simulink model "fsm_12B_with_contracts_SLDV"  (R2019b)
settings: Solver=FixedStepDiscrete  StartTime=0.0  StopTime=10  RelTol=1e-3  EnableMultiTasking=on
model workspace (MAT data in the model file):
  ContractValidatorBlocksMap : containers.Map (value not decoded)
libraries: sldvlib x20, cocosimLibs x20
(part 1 of 2)
settings Model: Creator=elliocm  LastModifiedBy=hbourbou
settings DataIOCC: LimitDataPoints=on  SaveFormat=Array  ReturnWorkspaceOutputs=off
settings OptimizationCC: ExpressionDepthLimit=2147483647  LifeSpan=inf
settings DebuggingCC: UnderspecifiedInitializationDetection=Classic  MergeDetectMultiDrivingBlocksExec=none  SolverPrmCheckMsg=warning  StateNameClashWarn=warning  SFUnexpectedBacktrackingDiag=warning  SFNoUnconditionalDefaultTransitionDiag=warning  SFExecutionAtInitializationDiag=none  ArithmeticOperatorsInVariantConditions=warning
settings HardwareCC: ProdBitPerPointer=32  ProdBitPerSizeT=32  ProdBitPerPtrDiffT=32  ProdLargestAtomicFloat=None  ProdIntDivRoundTo=Undefined  ProdEndianess=Unspecified  ProdWordSize=32  ProdHWDeviceType=32-bit Generic
settings ModelReferenceCC: PropagateSignalLabelsOutOfModel=off
settings SFSimCC: SimUseLocalCustomCode=off  CustomCodeUndefinedFunction=UseInterfaceOnly
settings RTWCC: RTWUseLocalCustomCode=off
settings CodeAppCC: StateflowObjectComments=on
settings GRTTargetCC: TargetLangStandard=C89/C90 (ANSI)  GeneratePreprocessorConditionals=Disable all
settings ConfigComp: CovMetricSettings=dw  CovHtmlReporting=on  CovSaveCumulativeToWorkspaceVar=on  CovSaveSingleToWorkspaceVar=on  CovExternalEMLEnable=off  DVMode=PropertyProving  DVTestSuiteOptimization=Auto  DVDetectOutOfBounds=on

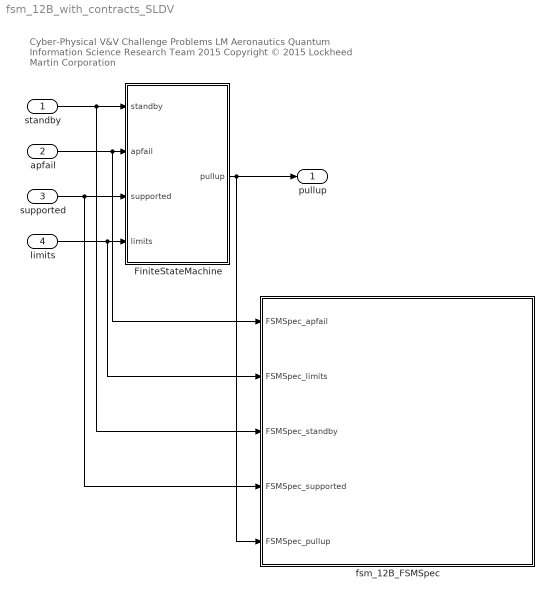
== system fsm_12B_with_contracts_SLDV ==
  note: Cyber-Physical V&V Challenge Problems
      | LM Aeronautics Quantum Information Science Research Team 2015
      | Copyright © 2015 Lockheed Martin Corporation
  standby : Inport  OutDataTypeStr=boolean
  apfail : Inport  Port=2  OutDataTypeStr=boolean
  supported : Inport  Port=3  OutDataTypeStr=boolean
  limits : Inport  Port=4  OutDataTypeStr=boolean
  FiniteStateMachine : Subsystem
  fsm_12B_FSMSpec : Subsystem  TreatAsAtomicUnit=on  SimViewingDevice=on  mask(VerificationSubsystem){}
      mask Display: image(imread('sldvicon_versubsys.png','BackGroundColor',[1 1 1]),'center');
  pullup : Outport  VectorParamsAs1DForOutWhenUnconnected=off
  wires:
  standby/1 -> FiniteStateMachine/1(standby), fsm_12B_FSMSpec/3(FSMSpec_standby)
  apfail/1 -> FiniteStateMachine/2(apfail), fsm_12B_FSMSpec/1(FSMSpec_apfail)
  supported/1 -> FiniteStateMachine/3(supported), fsm_12B_FSMSpec/4(FSMSpec_supported)
  limits/1 -> FiniteStateMachine/4(limits), fsm_12B_FSMSpec/2(FSMSpec_limits)
  FiniteStateMachine/1(pullup) -> pullup/1, fsm_12B_FSMSpec/5(FSMSpec_pullup)

== system fsm_12B_with_contracts_SLDV/FiniteStateMachine ==
  note: 51
  standby : Inport
  apfail : Inport  Port=2
  supported : Inport  Port=3
  limits : Inport  Port=4
  FiniteStateMachine_FSM_AutopilotSpec1 : Subsystem  TreatAsAtomicUnit=on  SimViewingDevice=on  mask(VerificationSubsystem){}
      mask Display: image(imread('sldvicon_versubsys.png','BackGroundColor',[1 1 1]),'center');
  FiniteStateMachine_FSM_SensorSpec : Subsystem  TreatAsAtomicUnit=on  SimViewingDevice=on  mask(VerificationSubsystem){}
      mask Display: image(imread('sldvicon_versubsys.png','BackGroundColor',[1 1 1]),'center');
  Manager : Subsystem
  Sen : Subsystem
  Unit Delay : UnitDelay  SampleTime=-1  HasFrameUpgradeWarning=on
  Unit Delay1 : UnitDelay  SampleTime=-1  HasFrameUpgradeWarning=on
  Unit Delay2 : UnitDelay  InitialCondition=1  SampleTime=-1  HasFrameUpgradeWarning=on
  pullup : Outport  VectorParamsAs1DForOutWhenUnconnected=off
  wires:
  Manager/1(MODE) -> FiniteStateMachine_FSM_SensorSpec/1(FSM_SensorSpec_MODE), Sen/1(mode)
  Manager/4(STATE) -> FiniteStateMachine_FSM_AutopilotSpec1/6(FSM_AutopilotSpec_STATE), Unit Delay/1
  Unit Delay/1 -> FiniteStateMachine_FSM_AutopilotSpec1/4(FSM_AutopilotSpec_state), Manager/5(state)
  Manager/2(REQUEST) -> FiniteStateMachine_FSM_SensorSpec/3(FSM_SensorSpec_request), Sen/2(request)
  Unit Delay1/1 -> FiniteStateMachine_FSM_SensorSpec/4(FSM_SensorSpec_senstate), Sen/4(senstate)
  Unit Delay2/1 -> FiniteStateMachine_FSM_AutopilotSpec1/2(FSM_AutopilotSpec_good), Manager/4(good)
  Sen/2(SENSTATE) -> FiniteStateMachine_FSM_SensorSpec/5(FSM_SensorSpec_SENSTATE), Unit Delay1/1
  Sen/1(good) -> Unit Delay2/1
  Manager/3(PULL) -> pullup/1
  standby/1 -> FiniteStateMachine_FSM_AutopilotSpec1/3(FSM_AutopilotSpec_standby), Manager/1(standby)
  apfail/1 -> FiniteStateMachine_FSM_AutopilotSpec1/1(FSM_AutopilotSpec_apfail), Manager/2(apfail)
  supported/1 -> FiniteStateMachine_FSM_AutopilotSpec1/5(FSM_AutopilotSpec_supported), Manager/3(supported)
  limits/1 -> Sen/3(limits), FiniteStateMachine_FSM_SensorSpec/2(FSM_SensorSpec_limits)

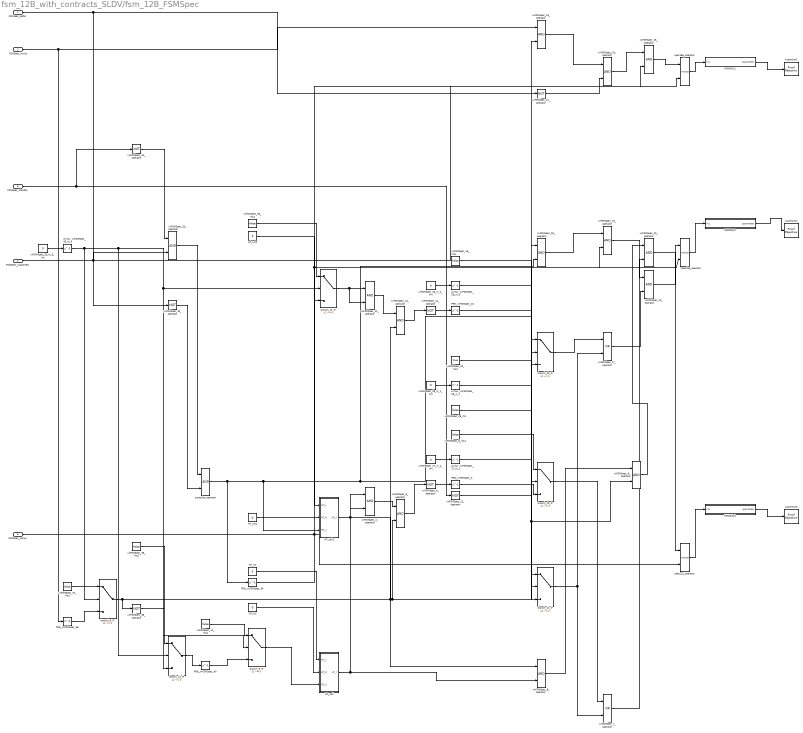
== system fsm_12B_with_contracts_SLDV/fsm_12B_FSMSpec ==
  FSMSpec_apfail : Inport  OutDataTypeStr=boolean
  FSMSpec_limits : Inport  Port=2  OutDataTypeStr=boolean
  FSMSpec_standby : Inport  Port=3  OutDataTypeStr=boolean
  FSMSpec_supported : Inport  Port=4  OutDataTypeStr=boolean
  FSMSpec_pullup : Inport  Port=5  OutDataTypeStr=boolean
  Arrow_xxFSMSpec_26_ni_0 : Delay  DelayLength=1  InitialCondition=1
  Arrow_xxFSMSpec_27_ni_2 : Delay  DelayLength=1  InitialCondition=1
  Arrow_xxFSMSpec_28_ni_1 : Delay  DelayLength=1  InitialCondition=1
  Arrow_xxFSMSpec_33_ni_5 : Delay  DelayLength=1  InitialCondition=1
  Assertion1 : sldvlib/Objectives and Constraints/Proof Objective  enabled=on  customAVTBlockType=Proof Objective  intervals=true  dispValues=on  outEnabled=off  enableStopSim=off
      settings: AttributesFormatString=%<intervals>  SourceProductName=Simulink  SourceProductBaseCode=SL
  Assertion2 : sldvlib/Objectives and Constraints/Proof Objective  enabled=on  customAVTBlockType=Proof Objective  intervals=true  dispValues=on  outEnabled=off  enableStopSim=off
      settings: AttributesFormatString=%<intervals>  SourceProductName=Simulink  SourceProductBaseCode=SL
  Assertion3 : sldvlib/Objectives and Constraints/Proof Objective  enabled=on  customAVTBlockType=Proof Objective  intervals=true  dispValues=on  outEnabled=off  enableStopSim=off
      settings: AttributesFormatString=%<intervals>  SourceProductName=Simulink  SourceProductBaseCode=SL
  FSM001v1 : Subsystem
  FSM001v2 : Subsystem
  FSM001v3 : Subsystem
  HT_In1 : Constant  Value=3  OutDataTypeStr=int32
  HT_In11 : Constant  Value=3  OutDataTypeStr=int32
  HT_In2 : Constant  Value=0  OutDataTypeStr=int32
  HT_In21 : Constant  Value=0  OutDataTypeStr=int32
  HT_call : Subsystem
  HT_call1 : Subsystem
  PRE_xxFSMSpec_{5,15,34,36,40} (5 alike) : Delay  DelayLength=1  InitialCondition=0
  autopilot_operator : Logic  AllPortsSameDT=off  OutDataTypeStr=boolean
  branch_10_IF : Switch  Criteria=u2 ~= 0
  branch_11_IF : Switch  Criteria=u2 ~= 0
  branch_12_IF : Switch  Criteria=u2 ~= 0
  branch_13_IF : Switch  Criteria=u2 ~= 0
  branch_14_IF : Switch  Criteria=u2 ~= 0
  branch_8_IF : Switch  Criteria=u2 ~= 0
  branch_9_IF : Switch  Criteria=u2 ~= 0
  spec166_operator : cocosimLibs/Implies  SystemSampleTime=-1  Latency=0  AutoFrameSizeCalculation=off
  spec194_operator : cocosimLibs/Implies  SystemSampleTime=-1  Latency=0  AutoFrameSizeCalculation=off
  spec222_operator : cocosimLibs/Implies  SystemSampleTime=-1  Latency=0  AutoFrameSizeCalculation=off
  xxFSMSpec_10_operator : Logic  AllPortsSameDT=off  OutDataTypeStr=boolean
  xxFSMSpec_12_operator : Logic  AllPortsSameDT=off  OutDataTypeStr=boolean
  xxFSMSpec_13_operator : Logic  AllPortsSameDT=off  OutDataTypeStr=boolean
  xxFSMSpec_14_operator : Logic  Operator=NOT  AllPortsSameDT=off  OutDataTypeStr=boolean
  xxFSMSpec_16_rhs1 : Constant  Value=false  OutDataTypeStr=boolean
  xxFSMSpec_17_operator : Logic  Operator=OR  AllPortsSameDT=off  OutDataTypeStr=boolean
  xxFSMSpec_18_operator : Logic  AllPortsSameDT=off  OutDataTypeStr=boolean
  xxFSMSpec_19_operator : Logic  AllPortsSameDT=off  OutDataTypeStr=boolean
  xxFSMSpec_20_operator : Logic  AllPortsSameDT=off  OutDataTypeStr=boolean
  xxFSMSpec_21_operator : Logic  Operator=NOT  AllPortsSameDT=off  OutDataTypeStr=boolean
  xxFSMSpec_22_operator : Logic  Operator=NOT  AllPortsSameDT=off  OutDataTypeStr=boolean
  xxFSMSpec_23_operator : Logic  AllPortsSameDT=off  OutDataTypeStr=boolean
  xxFSMSpec_24_operator : Logic  AllPortsSameDT=off  OutDataTypeStr=boolean
  xxFSMSpec_25_operator : Logic  AllPortsSameDT=off  OutDataTypeStr=boolean
  xxFSMSpec_26_ni_0_init : Constant  Value=0  OutDataTypeStr=boolean
  xxFSMSpec_27_ni_2_init : Constant  Value=0  OutDataTypeStr=boolean
  xxFSMSpec_28_ni_1_init : Constant  Value=0  OutDataTypeStr=boolean
  xxFSMSpec_29_rhs : Constant  Value=false  OutDataTypeStr=boolean
  xxFSMSpec_29_rhs1 : Constant  Value=true  OutDataTypeStr=boolean
  xxFSMSpec_2_operator : Logic  AllPortsSameDT=off  OutDataTypeStr=boolean
  xxFSMSpec_30_operator : Logic  Operator=NOT  AllPortsSameDT=off  OutDataTypeStr=boolean
  xxFSMSpec_31_operator : Logic  Operator=NOT  AllPortsSameDT=off  OutDataTypeStr=boolean
  xxFSMSpec_32_operator : Logic  AllPortsSameDT=off  OutDataTypeStr=boolean
  xxFSMSpec_33_ni_5_init : Constant  Value=0  OutDataTypeStr=boolean
  xxFSMSpec_35_rhs1 : Constant  Value=false  OutDataTypeStr=boolean
  xxFSMSpec_37_rhs1 : Constant  Value=false  OutDataTypeStr=boolean
  xxFSMSpec_38_operator : Logic  Operator=NOT  AllPortsSameDT=off  OutDataTypeStr=boolean
  xxFSMSpec_39_rhs1 : Constant  Value=false  OutDataTypeStr=boolean
  xxFSMSpec_3_operator : Logic  AllPortsSameDT=off  OutDataTypeStr=boolean
  xxFSMSpec_41_rhs1 : Constant  Value=false  OutDataTypeStr=boolean
  xxFSMSpec_4_operator : Logic  Operator=NOT  AllPortsSameDT=off  OutDataTypeStr=boolean
  xxFSMSpec_6_rhs1 : Constant  Value=false  OutDataTypeStr=boolean
  xxFSMSpec_7_operator : Logic  Operator=OR  AllPortsSameDT=off  OutDataTypeStr=boolean
  xxFSMSpec_8_operator : Logic  AllPortsSameDT=off  OutDataTypeStr=boolean
  xxFSMSpec_9_operator : Logic  AllPortsSameDT=off  OutDataTypeStr=boolean
  wires:
  xxFSMSpec_8_operator/1 -> xxFSMSpec_9_operator/1
  branch_10_IF/1 -> xxFSMSpec_7_operator/1
  xxFSMSpec_3_operator/1 -> xxFSMSpec_4_operator/1
  xxFSMSpec_2_operator/1 -> xxFSMSpec_3_operator/1
  xxFSMSpec_31_operator/1 -> xxFSMSpec_32_operator/1
  xxFSMSpec_24_operator/1 -> xxFSMSpec_25_operator/1
  xxFSMSpec_21_operator/1 -> xxFSMSpec_24_operator/2
  xxFSMSpec_23_operator/1 -> xxFSMSpec_24_operator/1
  xxFSMSpec_22_operator/1 -> xxFSMSpec_23_operator/2
  xxFSMSpec_17_operator/1 -> xxFSMSpec_20_operator/2
  xxFSMSpec_19_operator/1 -> xxFSMSpec_20_operator/1
  xxFSMSpec_18_operator/1 -> xxFSMSpec_19_operator/1
  branch_13_IF/1 -> xxFSMSpec_17_operator/1
  xxFSMSpec_13_operator/1 -> xxFSMSpec_14_operator/1
  xxFSMSpec_12_operator/1 -> xxFSMSpec_13_operator/1
  xxFSMSpec_7_operator/1 -> xxFSMSpec_10_operator/2
  xxFSMSpec_9_operator/1 -> xxFSMSpec_10_operator/1
  xxFSMSpec_10_operator/1 -> spec222_operator/1
  xxFSMSpec_20_operator/1 -> spec194_operator/1
  xxFSMSpec_25_operator/1 -> spec166_operator/1
  spec222_operator/1 -> FSM001v3/1(In1)
  spec194_operator/1 -> FSM001v2/1(In1)
  spec166_operator/1 -> FSM001v1/1(In1)
  PRE_xxFSMSpec_40/1 -> branch_9_IF/3
  xxFSMSpec_41_rhs1/1 -> branch_9_IF/1
  PRE_xxFSMSpec_36/1 -> branch_8_IF/3
  xxFSMSpec_37_rhs1/1 -> branch_8_IF/1
  xxFSMSpec_38_operator/1 -> branch_14_IF/3
  xxFSMSpec_39_rhs1/1 -> branch_14_IF/1
  PRE_xxFSMSpec_15/1 -> branch_13_IF/3
  Arrow_xxFSMSpec_26_ni_0/1 -> branch_13_IF/2
  xxFSMSpec_16_rhs1/1 -> branch_13_IF/1
  PRE_xxFSMSpec_34/1 -> branch_12_IF/3
  xxFSMSpec_35_rhs1/1 -> branch_12_IF/1
  xxFSMSpec_29_rhs/1 -> branch_11_IF/3
  Arrow_xxFSMSpec_28_ni_1/1 -> branch_11_IF/2
  xxFSMSpec_29_rhs1/1 -> branch_11_IF/1
  PRE_xxFSMSpec_5/1 -> branch_10_IF/3
  Arrow_xxFSMSpec_27_ni_2/1 -> branch_10_IF/2
  xxFSMSpec_6_rhs1/1 -> branch_10_IF/1
  xxFSMSpec_30_operator/1 -> autopilot_operator/2
  xxFSMSpec_32_operator/1 -> autopilot_operator/1
  xxFSMSpec_4_operator/1 -> PRE_xxFSMSpec_5/1
  branch_14_IF/1 -> PRE_xxFSMSpec_40/1
  xxFSMSpec_14_operator/1 -> PRE_xxFSMSpec_15/1
  HT_In21/1 -> HT_call1/2(HT_R)
  HT_In11/1 -> HT_call1/1(HT_L)
  branch_9_IF/1 -> HT_call/3(HT_X)
  HT_In2/1 -> HT_call/2(HT_R)
  HT_In1/1 -> HT_call/1(HT_L)
  xxFSMSpec_33_ni_5_init/1 -> Arrow_xxFSMSpec_33_ni_5/1
  xxFSMSpec_28_ni_1_init/1 -> Arrow_xxFSMSpec_28_ni_1/1
  xxFSMSpec_27_ni_2_init/1 -> Arrow_xxFSMSpec_27_ni_2/1
  xxFSMSpec_26_ni_0_init/1 -> Arrow_xxFSMSpec_26_ni_0/1
  branch_8_IF/1 -> xxFSMSpec_9_operator/2, xxFSMSpec_19_operator/2, xxFSMSpec_3_operator/2, xxFSMSpec_13_operator/2, xxFSMSpec_38_operator/1
  branch_12_IF/1 -> xxFSMSpec_18_operator/2, xxFSMSpec_12_operator/2
  HT_call/1(HT_Y) -> xxFSMSpec_8_operator/2, xxFSMSpec_2_operator/2
  HT_call1/1(HT_Y) -> xxFSMSpec_8_operator/1, xxFSMSpec_2_operator/1
  FSMSpec_pullup/1 -> spec194_operator/2, spec166_operator/2, spec222_operator/2
  FSMSpec_supported/1 -> xxFSMSpec_32_operator/2, xxFSMSpec_25_operator/2
  FSMSpec_apfail/1 -> xxFSMSpec_30_operator/1, xxFSMSpec_21_operator/1
  FSMSpec_limits/1 -> xxFSMSpec_23_operator/1, PRE_xxFSMSpec_36/1
  FSMSpec_standby/1 -> xxFSMSpec_31_operator/1, xxFSMSpec_22_operator/1
  branch_11_IF/1 -> xxFSMSpec_7_operator/2, xxFSMSpec_17_operator/2
  Arrow_xxFSMSpec_33_ni_5/1 -> branch_9_IF/2, branch_12_IF/2, branch_14_IF/2, branch_8_IF/2
  autopilot_operator/1 -> xxFSMSpec_18_operator/1, xxFSMSpec_12_operator/1, HT_call1/3(HT_X), PRE_xxFSMSpec_34/1
  FSM001v1/1(guarantee) -> Assertion1/1
  FSM001v2/1(guarantee) -> Assertion2/1
  FSM001v3/1(guarantee) -> Assertion3/1

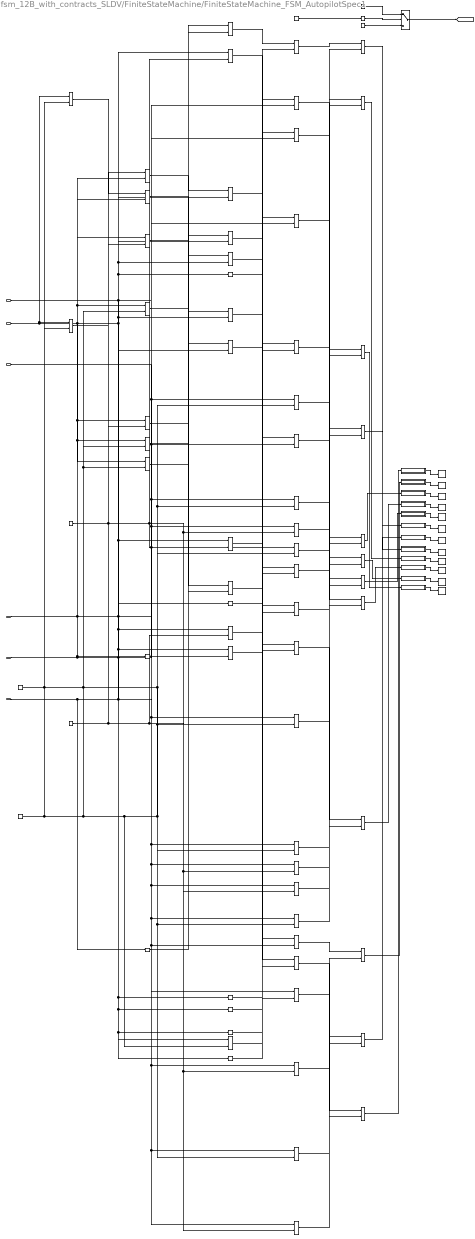
== system fsm_12B_with_contracts_SLDV/FiniteStateMachine/FiniteStateMachine_FSM_AutopilotSpec1 ==
  FSM_AutopilotSpec_apfail : Inport  OutDataTypeStr=boolean
  FSM_AutopilotSpec_good : Inport  Port=2  OutDataTypeStr=boolean
  FSM_AutopilotSpec_standby : Inport  Port=3  OutDataTypeStr=boolean
  FSM_AutopilotSpec_state : Inport  Port=4  OutDataTypeStr=double
  FSM_AutopilotSpec_supported : Inport  Port=5  OutDataTypeStr=boolean
  FSM_AutopilotSpec_STATE : Inport  Port=6  OutDataTypeStr=double
  Arrow_xxFSM_AutopilotSpec_54_ni_7 : Delay  DelayLength=1  InitialCondition=1
  Assertion{1..12} (12 alike) : sldvlib/Objectives and Constraints/Proof Objective  enabled=on  customAVTBlockType=Proof Objective  intervals=true  dispValues=on  outEnabled=off  enableStopSim=off
      settings: AttributesFormatString=%<intervals>  SourceProductName=Simulink  SourceProductBaseCode=SL
  FSM002 : Subsystem
  FSM003 : Subsystem
  FSM003v2 : Subsystem
  FSM004 : Subsystem
  FSM004v2 : Subsystem
  FSM005 : Subsystem
  FSM006 : Subsystem
  FSM007 : Subsystem
  FSM007v2 : Subsystem
  FSM008v1 : Subsystem
  FSM008v2 : Subsystem
  FSM009 : Subsystem
  branch_6_IF : Switch  Criteria=u2 ~= 0
  spec129_operator : cocosimLibs/Implies  SystemSampleTime=-1  Latency=0  AutoFrameSizeCalculation=off
  spec143_operator : cocosimLibs/Implies  SystemSampleTime=-1  Latency=0  AutoFrameSizeCalculation=off
  spec160_operator : cocosimLibs/Implies  SystemSampleTime=-1  Latency=0  AutoFrameSizeCalculation=off
  spec182_operator : cocosimLibs/Implies  SystemSampleTime=-1  Latency=0  AutoFrameSizeCalculation=off
  spec198_operator : cocosimLibs/Implies  SystemSampleTime=-1  Latency=0  AutoFrameSizeCalculation=off
  spec212_operator : cocosimLibs/Implies  SystemSampleTime=-1  Latency=0  AutoFrameSizeCalculation=off
  spec233_operator : cocosimLibs/Implies  SystemSampleTime=-1  Latency=0  AutoFrameSizeCalculation=off
  spec254_operator : cocosimLibs/Implies  SystemSampleTime=-1  Latency=0  AutoFrameSizeCalculation=off
  spec271_operator : cocosimLibs/Implies  SystemSampleTime=-1  Latency=0  AutoFrameSizeCalculation=off
  spec287_operator : cocosimLibs/Implies  SystemSampleTime=-1  Latency=0  AutoFrameSizeCalculation=off
  spec309_operator : cocosimLibs/Implies  SystemSampleTime=-1  Latency=0  AutoFrameSizeCalculation=off
  spec326_operator : cocosimLibs/Implies  SystemSampleTime=-1  Latency=0  AutoFrameSizeCalculation=off
  xxFSM_AutopilotSpec_10_operator : Logic  AllPortsSameDT=off  OutDataTypeStr=boolean
  xxFSM_AutopilotSpec_11_operator : RelationalOperator  Operator===  OutDataTypeStr=boolean  RndMeth=Simplest
  xxFSM_AutopilotSpec_12_operator : RelationalOperator  Operator===  OutDataTypeStr=boolean  RndMeth=Simplest
  xxFSM_AutopilotSpec_13_operator : Logic  Operator=NOT  AllPortsSameDT=off  OutDataTypeStr=boolean
  xxFSM_AutopilotSpec_14_operator : Logic  AllPortsSameDT=off  OutDataTypeStr=boolean
  xxFSM_AutopilotSpec_15_operator : RelationalOperator  Operator===  OutDataTypeStr=boolean  RndMeth=Simplest
  xxFSM_AutopilotSpec_16_operator : RelationalOperator  Operator===  OutDataTypeStr=boolean  RndMeth=Simplest
  xxFSM_AutopilotSpec_17_operator : Logic  AllPortsSameDT=off  OutDataTypeStr=boolean
  xxFSM_AutopilotSpec_18_operator : Logic  AllPortsSameDT=off  OutDataTypeStr=boolean
  xxFSM_AutopilotSpec_19_operator : RelationalOperator  Operator===  OutDataTypeStr=boolean  RndMeth=Simplest
  xxFSM_AutopilotSpec_1_operator : RelationalOperator  Operator===  OutDataTypeStr=boolean  RndMeth=Simplest
  xxFSM_AutopilotSpec_20_operator : Logic  Operator=NOT  AllPortsSameDT=off  OutDataTypeStr=boolean
  xxFSM_AutopilotSpec_21_operator : Logic  Operator=NOT  AllPortsSameDT=off  OutDataTypeStr=boolean
  xxFSM_AutopilotSpec_22_operator : RelationalOperator  Operator===  OutDataTypeStr=boolean  RndMeth=Simplest
  xxFSM_AutopilotSpec_23_operator : Logic  AllPortsSameDT=off  OutDataTypeStr=boolean
  xxFSM_AutopilotSpec_24_operator : Logic  AllPortsSameDT=off  OutDataTypeStr=boolean
  xxFSM_AutopilotSpec_25_operator : RelationalOperator  Operator===  OutDataTypeStr=boolean  RndMeth=Simplest
  xxFSM_AutopilotSpec_26_operator : Logic  Operator=NOT  AllPortsSameDT=off  OutDataTypeStr=boolean
  xxFSM_AutopilotSpec_27_operator : Logic  Operator=NOT  AllPortsSameDT=off  OutDataTypeStr=boolean
  xxFSM_AutopilotSpec_28_operator : RelationalOperator  Operator===  OutDataTypeStr=boolean  RndMeth=Simplest
  xxFSM_AutopilotSpec_29_operator : Logic  AllPortsSameDT=off  OutDataTypeStr=boolean
  xxFSM_AutopilotSpec_2_operator : RelationalOperator  Operator===  OutDataTypeStr=boolean  RndMeth=Simplest
  xxFSM_AutopilotSpec_30_operator : Logic  AllPortsSameDT=off  OutDataTypeStr=boolean
  xxFSM_AutopilotSpec_31_operator : RelationalOperator  Operator===  OutDataTypeStr=boolean  RndMeth=Simplest
  xxFSM_AutopilotSpec_32_operator : RelationalOperator  Operator===  OutDataTypeStr=boolean  RndMeth=Simplest
  xxFSM_AutopilotSpec_33_operator : Logic  AllPortsSameDT=off  OutDataTypeStr=boolean
  xxFSM_AutopilotSpec_34_operator : RelationalOperator  Operator===  OutDataTypeStr=boolean  RndMeth=Simplest
  xxFSM_AutopilotSpec_35_operator : Logic  Operator=NOT  AllPortsSameDT=off  OutDataTypeStr=boolean
  xxFSM_AutopilotSpec_36_operator : RelationalOperator  Operator===  OutDataTypeStr=boolean  RndMeth=Simplest
  xxFSM_AutopilotSpec_37_operator : Logic  AllPortsSameDT=off  OutDataTypeStr=boolean
  xxFSM_AutopilotSpec_38_operator : RelationalOperator  Operator===  OutDataTypeStr=boolean  RndMeth=Simplest
  xxFSM_AutopilotSpec_39_operator : Logic  Operator=NOT  AllPortsSameDT=off  OutDataTypeStr=boolean
  xxFSM_AutopilotSpec_3_operator : Logic  AllPortsSameDT=off  OutDataTypeStr=boolean
  xxFSM_AutopilotSpec_40_operator : RelationalOperator  Operator===  OutDataTypeStr=boolean  RndMeth=Simplest
  xxFSM_AutopilotSpec_41_operator : Logic  AllPortsSameDT=off  OutDataTypeStr=boolean
  xxFSM_AutopilotSpec_42_operator : Logic  AllPortsSameDT=off  OutDataTypeStr=boolean
  xxFSM_AutopilotSpec_43_operator : Logic  AllPortsSameDT=off  OutDataTypeStr=boolean
  xxFSM_AutopilotSpec_44_operator : RelationalOperator  Operator===  OutDataTypeStr=boolean  RndMeth=Simplest
  xxFSM_AutopilotSpec_45_operator : RelationalOperator  Operator===  OutDataTypeStr=boolean  RndMeth=Simplest
  xxFSM_AutopilotSpec_46_operator : Logic  AllPortsSameDT=off  OutDataTypeStr=boolean
  xxFSM_AutopilotSpec_47_operator : Logic  AllPortsSameDT=off  OutDataTypeStr=boolean
  xxFSM_AutopilotSpec_48_operator : RelationalOperator  Operator===  OutDataTypeStr=boolean  RndMeth=Simplest
  xxFSM_AutopilotSpec_49_operator : RelationalOperator  Operator===  OutDataTypeStr=boolean  RndMeth=Simplest
  xxFSM_AutopilotSpec_4_operator : Logic  AllPortsSameDT=off  OutDataTypeStr=boolean
  xxFSM_AutopilotSpec_50_operator : Logic  AllPortsSameDT=off  OutDataTypeStr=boolean
  xxFSM_AutopilotSpec_51_operator : RelationalOperator  Operator===  OutDataTypeStr=boolean  RndMeth=Simplest
  xxFSM_AutopilotSpec_52_operator : RelationalOperator  Operator===  OutDataTypeStr=boolean  RndMeth=Simplest
  xxFSM_AutopilotSpec_53_operator : Logic  AllPortsSameDT=off  OutDataTypeStr=boolean
  xxFSM_AutopilotSpec_54_ni_7_init : Constant  Value=0  OutDataTypeStr=boolean
  xxFSM_AutopilotSpec_55_rhs : Constant  Value=false  OutDataTypeStr=boolean
  xxFSM_AutopilotSpec_55_rhs1 : Constant  Value=true  OutDataTypeStr=boolean
  xxFSM_AutopilotSpec_56_rhs : Constant  Value=2.0  OutDataTypeStr=double
  xxFSM_AutopilotSpec_57_rhs : Constant  Value=1.0  OutDataTypeStr=double
  xxFSM_AutopilotSpec_58_rhs : Constant  Value=3.0  OutDataTypeStr=double
  xxFSM_AutopilotSpec_59_rhs : Constant  Value=0.0  OutDataTypeStr=double
  xxFSM_AutopilotSpec_5_operator : RelationalOperator  Operator===  OutDataTypeStr=boolean  RndMeth=Simplest
  xxFSM_AutopilotSpec_6_operator : Logic  Operator=NOT  AllPortsSameDT=off  OutDataTypeStr=boolean
  xxFSM_AutopilotSpec_7_operator : RelationalOperator  Operator===  OutDataTypeStr=boolean  RndMeth=Simplest
  xxFSM_AutopilotSpec_8_operator : Logic  AllPortsSameDT=off  OutDataTypeStr=boolean
  xxFSM_AutopilotSpec_9_operator : Logic  AllPortsSameDT=off  OutDataTypeStr=boolean
  wires:
  xxFSM_AutopilotSpec_8_operator/1 -> xxFSM_AutopilotSpec_9_operator/1
  xxFSM_AutopilotSpec_7_operator/1 -> xxFSM_AutopilotSpec_8_operator/1
  xxFSM_AutopilotSpec_52_operator/1 -> xxFSM_AutopilotSpec_53_operator/2
  xxFSM_AutopilotSpec_49_operator/1 -> xxFSM_AutopilotSpec_50_operator/1
  xxFSM_AutopilotSpec_3_operator/1 -> xxFSM_AutopilotSpec_4_operator/1
  xxFSM_AutopilotSpec_46_operator/1 -> xxFSM_AutopilotSpec_47_operator/1
  xxFSM_AutopilotSpec_45_operator/1 -> xxFSM_AutopilotSpec_46_operator/1
  xxFSM_AutopilotSpec_39_operator/1 -> xxFSM_AutopilotSpec_43_operator/2
  xxFSM_AutopilotSpec_42_operator/1 -> xxFSM_AutopilotSpec_43_operator/1
  xxFSM_AutopilotSpec_41_operator/1 -> xxFSM_AutopilotSpec_42_operator/1
  xxFSM_AutopilotSpec_40_operator/1 -> xxFSM_AutopilotSpec_41_operator/1
  xxFSM_AutopilotSpec_2_operator/1 -> xxFSM_AutopilotSpec_3_operator/1
  xxFSM_AutopilotSpec_35_operator/1 -> xxFSM_AutopilotSpec_37_operator/2
  xxFSM_AutopilotSpec_36_operator/1 -> xxFSM_AutopilotSpec_37_operator/1
  xxFSM_AutopilotSpec_32_operator/1 -> xxFSM_AutopilotSpec_33_operator/1
  xxFSM_AutopilotSpec_26_operator/1 -> xxFSM_AutopilotSpec_30_operator/2
  xxFSM_AutopilotSpec_29_operator/1 -> xxFSM_AutopilotSpec_30_operator/1
  xxFSM_AutopilotSpec_27_operator/1 -> xxFSM_AutopilotSpec_29_operator/2
  xxFSM_AutopilotSpec_28_operator/1 -> xxFSM_AutopilotSpec_29_operator/1
  xxFSM_AutopilotSpec_20_operator/1 -> xxFSM_AutopilotSpec_24_operator/2
  xxFSM_AutopilotSpec_23_operator/1 -> xxFSM_AutopilotSpec_24_operator/1
  xxFSM_AutopilotSpec_21_operator/1 -> xxFSM_AutopilotSpec_23_operator/2
  xxFSM_AutopilotSpec_22_operator/1 -> xxFSM_AutopilotSpec_23_operator/1
  xxFSM_AutopilotSpec_17_operator/1 -> xxFSM_AutopilotSpec_18_operator/1
  xxFSM_AutopilotSpec_16_operator/1 -> xxFSM_AutopilotSpec_17_operator/1
  xxFSM_AutopilotSpec_12_operator/1 -> xxFSM_AutopilotSpec_14_operator/2
  xxFSM_AutopilotSpec_13_operator/1 -> xxFSM_AutopilotSpec_14_operator/1
  xxFSM_AutopilotSpec_6_operator/1 -> xxFSM_AutopilotSpec_10_operator/2
  xxFSM_AutopilotSpec_9_operator/1 -> xxFSM_AutopilotSpec_10_operator/1
  xxFSM_AutopilotSpec_1_operator/1 -> spec326_operator/2
  xxFSM_AutopilotSpec_4_operator/1 -> spec326_operator/1
  xxFSM_AutopilotSpec_5_operator/1 -> spec309_operator/2
  xxFSM_AutopilotSpec_10_operator/1 -> spec309_operator/1
  xxFSM_AutopilotSpec_11_operator/1 -> spec287_operator/2
  xxFSM_AutopilotSpec_14_operator/1 -> spec287_operator/1
  xxFSM_AutopilotSpec_15_operator/1 -> spec271_operator/2
  xxFSM_AutopilotSpec_18_operator/1 -> spec271_operator/1
  xxFSM_AutopilotSpec_19_operator/1 -> spec254_operator/2
  xxFSM_AutopilotSpec_24_operator/1 -> spec254_operator/1
  xxFSM_AutopilotSpec_25_operator/1 -> spec233_operator/2
  xxFSM_AutopilotSpec_30_operator/1 -> spec233_operator/1
  xxFSM_AutopilotSpec_31_operator/1 -> spec212_operator/2
  xxFSM_AutopilotSpec_33_operator/1 -> spec212_operator/1
  xxFSM_AutopilotSpec_34_operator/1 -> spec198_operator/2
  xxFSM_AutopilotSpec_37_operator/1 -> spec198_operator/1
  xxFSM_AutopilotSpec_38_operator/1 -> spec182_operator/2
  xxFSM_AutopilotSpec_43_operator/1 -> spec182_operator/1
  xxFSM_AutopilotSpec_44_operator/1 -> spec160_operator/2
  xxFSM_AutopilotSpec_47_operator/1 -> spec160_operator/1
  xxFSM_AutopilotSpec_48_operator/1 -> spec143_operator/2
  xxFSM_AutopilotSpec_50_operator/1 -> spec143_operator/1
  xxFSM_AutopilotSpec_51_operator/1 -> spec129_operator/2
  xxFSM_AutopilotSpec_53_operator/1 -> spec129_operator/1
  spec326_operator/1 -> FSM006/1(In1)
  spec309_operator/1 -> FSM007v2/1(In1)
  spec287_operator/1 -> FSM004/1(In1)
  spec271_operator/1 -> FSM007/1(In1)
  spec254_operator/1 -> FSM008v2/1(In1)
  spec233_operator/1 -> FSM004v2/1(In1)
  spec212_operator/1 -> FSM009/1(In1)
  spec198_operator/1 -> FSM008v1/1(In1)
  spec182_operator/1 -> FSM003v2/1(In1)
  spec160_operator/1 -> FSM003/1(In1)
  spec143_operator/1 -> FSM005/1(In1)
  spec129_operator/1 -> FSM002/1(In1)
  xxFSM_AutopilotSpec_55_rhs/1 -> branch_6_IF/3
  Arrow_xxFSM_AutopilotSpec_54_ni_7/1 -> branch_6_IF/2
  xxFSM_AutopilotSpec_55_rhs1/1 -> branch_6_IF/1
  branch_6_IF/1 -> [FSM_AutopilotSpec_FTP]
  xxFSM_AutopilotSpec_54_ni_7_init/1 -> Arrow_xxFSM_AutopilotSpec_54_ni_7/1
  FSM_AutopilotSpec_apfail/1 -> xxFSM_AutopilotSpec_33_operator/2, xxFSM_AutopilotSpec_20_operator/1
  FSM_AutopilotSpec_standby/1 -> xxFSM_AutopilotSpec_6_operator/1, xxFSM_AutopilotSpec_26_operator/1, xxFSM_AutopilotSpec_35_operator/1, xxFSM_AutopilotSpec_39_operator/1, xxFSM_AutopilotSpec_53_operator/1, xxFSM_AutopilotSpec_50_operator/2, xxFSM_AutopilotSpec_3_operator/2, xxFSM_AutopilotSpec_21_operator/1
  xxFSM_AutopilotSpec_59_rhs/1 -> xxFSM_AutopilotSpec_19_operator/2, xxFSM_AutopilotSpec_15_operator/2, xxFSM_AutopilotSpec_5_operator/2, xxFSM_AutopilotSpec_34_operator/2, xxFSM_AutopilotSpec_52_operator/2, xxFSM_AutopilotSpec_45_operator/2, xxFSM_AutopilotSpec_40_operator/2
  FSM_AutopilotSpec_supported/1 -> xxFSM_AutopilotSpec_42_operator/2, xxFSM_AutopilotSpec_17_operator/2, xxFSM_AutopilotSpec_47_operator/2, xxFSM_AutopilotSpec_8_operator/2
  xxFSM_AutopilotSpec_56_rhs/1 -> xxFSM_AutopilotSpec_25_operator/2, xxFSM_AutopilotSpec_11_operator/2, xxFSM_AutopilotSpec_31_operator/2, xxFSM_AutopilotSpec_2_operator/2, xxFSM_AutopilotSpec_16_operator/2, xxFSM_AutopilotSpec_7_operator/2
  FSM_AutopilotSpec_STATE/1 -> xxFSM_AutopilotSpec_51_operator/1, xxFSM_AutopilotSpec_25_operator/1, xxFSM_AutopilotSpec_48_operator/1, xxFSM_AutopilotSpec_11_operator/1, xxFSM_AutopilotSpec_44_operator/1, xxFSM_AutopilotSpec_38_operator/1, xxFSM_AutopilotSpec_34_operator/1, xxFSM_AutopilotSpec_5_operator/1, xxFSM_AutopilotSpec_31_operator/1, xxFSM_AutopilotSpec_1_operator/1, xxFSM_AutopilotSpec_15_operator/1, xxFSM_AutopilotSpec_19_operator/1
  xxFSM_AutopilotSpec_57_rhs/1 -> xxFSM_AutopilotSpec_44_operator/2, xxFSM_AutopilotSpec_38_operator/2, xxFSM_AutopilotSpec_49_operator/2, xxFSM_AutopilotSpec_12_operator/2, xxFSM_AutopilotSpec_28_operator/2
  FSM_AutopilotSpec_state/1 -> xxFSM_AutopilotSpec_2_operator/1, xxFSM_AutopilotSpec_16_operator/1, xxFSM_AutopilotSpec_22_operator/1, xxFSM_AutopilotSpec_52_operator/1, xxFSM_AutopilotSpec_12_operator/1, xxFSM_AutopilotSpec_49_operator/1, xxFSM_AutopilotSpec_36_operator/1, xxFSM_AutopilotSpec_32_operator/1, xxFSM_AutopilotSpec_45_operator/1, xxFSM_AutopilotSpec_28_operator/1, xxFSM_AutopilotSpec_7_operator/1, xxFSM_AutopilotSpec_40_operator/1
  FSM_AutopilotSpec_good/1 -> xxFSM_AutopilotSpec_4_operator/2, xxFSM_AutopilotSpec_18_operator/2, xxFSM_AutopilotSpec_46_operator/2, xxFSM_AutopilotSpec_13_operator/1, xxFSM_AutopilotSpec_9_operator/2, xxFSM_AutopilotSpec_41_operator/2, xxFSM_AutopilotSpec_27_operator/1
  xxFSM_AutopilotSpec_58_rhs/1 -> xxFSM_AutopilotSpec_51_operator/2, xxFSM_AutopilotSpec_48_operator/2, xxFSM_AutopilotSpec_1_operator/2, xxFSM_AutopilotSpec_36_operator/2, xxFSM_AutopilotSpec_32_operator/2, xxFSM_AutopilotSpec_22_operator/2
  FSM002/1(guarantee) -> Assertion1/1
  FSM005/1(guarantee) -> Assertion2/1
  FSM003/1(guarantee) -> Assertion3/1
  FSM003v2/1(guarantee) -> Assertion4/1
  FSM008v1/1(guarantee) -> Assertion5/1
  FSM009/1(guarantee) -> Assertion6/1
  FSM004v2/1(guarantee) -> Assertion7/1
  FSM008v2/1(guarantee) -> Assertion8/1
  FSM007/1(guarantee) -> Assertion9/1
  FSM004/1(guarantee) -> Assertion10/1
  FSM007v2/1(guarantee) -> Assertion11/1
  FSM006/1(guarantee) -> Assertion12/1

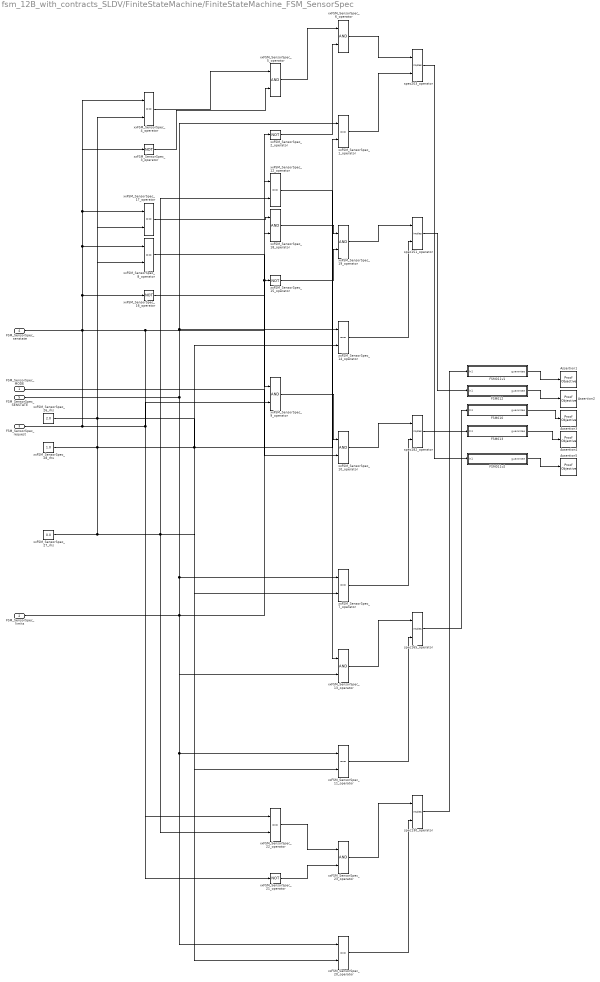
== system fsm_12B_with_contracts_SLDV/FiniteStateMachine/FiniteStateMachine_FSM_SensorSpec ==
  FSM_SensorSpec_MODE : Inport  OutDataTypeStr=boolean
  FSM_SensorSpec_limits : Inport  Port=2  OutDataTypeStr=boolean
  FSM_SensorSpec_request : Inport  Port=3  OutDataTypeStr=boolean
  FSM_SensorSpec_senstate : Inport  Port=4  OutDataTypeStr=double
  FSM_SensorSpec_SENSTATE : Inport  Port=5  OutDataTypeStr=double
  Assertion{1..5} (5 alike) : sldvlib/Objectives and Constraints/Proof Objective  enabled=on  customAVTBlockType=Proof Objective  intervals=true  dispValues=on  outEnabled=off  enableStopSim=off
      settings: AttributesFormatString=%<intervals>  SourceProductName=Simulink  SourceProductBaseCode=SL
  FSM010 : Subsystem
  FSM011v1 : Subsystem
  FSM011v2 : Subsystem
  FSM012 : Subsystem
  FSM013 : Subsystem
  spec130_operator : cocosimLibs/Implies  SystemSampleTime=-1  Latency=0  AutoFrameSizeCalculation=off
  spec151_operator : cocosimLibs/Implies  SystemSampleTime=-1  Latency=0  AutoFrameSizeCalculation=off
  spec165_operator : cocosimLibs/Implies  SystemSampleTime=-1  Latency=0  AutoFrameSizeCalculation=off
  spec182_operator : cocosimLibs/Implies  SystemSampleTime=-1  Latency=0  AutoFrameSizeCalculation=off
  spec203_operator : cocosimLibs/Implies  SystemSampleTime=-1  Latency=0  AutoFrameSizeCalculation=off
  xxFSM_SensorSpec_10_operator : Logic  AllPortsSameDT=off  OutDataTypeStr=boolean
  xxFSM_SensorSpec_11_operator : RelationalOperator  Operator===  OutDataTypeStr=boolean  RndMeth=Simplest
  xxFSM_SensorSpec_12_operator : RelationalOperator  Operator===  OutDataTypeStr=boolean  RndMeth=Simplest
  xxFSM_SensorSpec_13_operator : Logic  AllPortsSameDT=off  OutDataTypeStr=boolean
  xxFSM_SensorSpec_14_operator : RelationalOperator  Operator===  OutDataTypeStr=boolean  RndMeth=Simplest
  xxFSM_SensorSpec_15_operator : Logic  Operator=NOT  AllPortsSameDT=off  OutDataTypeStr=boolean
  xxFSM_SensorSpec_16_operator : Logic  Operator=NOT  AllPortsSameDT=off  OutDataTypeStr=boolean
  xxFSM_SensorSpec_17_operator : RelationalOperator  Operator===  OutDataTypeStr=boolean  RndMeth=Simplest
  xxFSM_SensorSpec_18_operator : Logic  AllPortsSameDT=off  OutDataTypeStr=boolean
  xxFSM_SensorSpec_19_operator : Logic  AllPortsSameDT=off  OutDataTypeStr=boolean
  xxFSM_SensorSpec_1_operator : RelationalOperator  Operator===  OutDataTypeStr=boolean  RndMeth=Simplest
  xxFSM_SensorSpec_20_operator : RelationalOperator  Operator===  OutDataTypeStr=boolean  RndMeth=Simplest
  xxFSM_SensorSpec_21_operator : Logic  Operator=NOT  AllPortsSameDT=off  OutDataTypeStr=boolean
  xxFSM_SensorSpec_22_operator : RelationalOperator  Operator===  OutDataTypeStr=boolean  RndMeth=Simplest
  xxFSM_SensorSpec_23_operator : Logic  AllPortsSameDT=off  OutDataTypeStr=boolean
  xxFSM_SensorSpec_26_rhs : Constant  Value=2.0  OutDataTypeStr=double
  xxFSM_SensorSpec_27_rhs : Constant  Value=0.0  OutDataTypeStr=double
  xxFSM_SensorSpec_28_rhs : Constant  Value=1.0  OutDataTypeStr=double
  xxFSM_SensorSpec_2_operator : Logic  Operator=NOT  AllPortsSameDT=off  OutDataTypeStr=boolean
  xxFSM_SensorSpec_3_operator : Logic  Operator=NOT  AllPortsSameDT=off  OutDataTypeStr=boolean
  xxFSM_SensorSpec_4_operator : RelationalOperator  Operator===  OutDataTypeStr=boolean  RndMeth=Simplest
  xxFSM_SensorSpec_5_operator : Logic  AllPortsSameDT=off  OutDataTypeStr=boolean
  xxFSM_SensorSpec_6_operator : Logic  AllPortsSameDT=off  OutDataTypeStr=boolean
  xxFSM_SensorSpec_7_operator : RelationalOperator  Operator===  OutDataTypeStr=boolean  RndMeth=Simplest
  xxFSM_SensorSpec_8_operator : RelationalOperator  Operator===  OutDataTypeStr=boolean  RndMeth=Simplest
  xxFSM_SensorSpec_9_operator : Logic  AllPortsSameDT=off  OutDataTypeStr=boolean
  wires:
  xxFSM_SensorSpec_8_operator/1 -> xxFSM_SensorSpec_9_operator/1
  xxFSM_SensorSpec_2_operator/1 -> xxFSM_SensorSpec_6_operator/2
  xxFSM_SensorSpec_5_operator/1 -> xxFSM_SensorSpec_6_operator/1
  xxFSM_SensorSpec_3_operator/1 -> xxFSM_SensorSpec_5_operator/2
  xxFSM_SensorSpec_4_operator/1 -> xxFSM_SensorSpec_5_operator/1
  xxFSM_SensorSpec_21_operator/1 -> xxFSM_SensorSpec_23_operator/2
  xxFSM_SensorSpec_22_operator/1 -> xxFSM_SensorSpec_23_operator/1
  xxFSM_SensorSpec_15_operator/1 -> xxFSM_SensorSpec_19_operator/2
  xxFSM_SensorSpec_18_operator/1 -> xxFSM_SensorSpec_19_operator/1
  xxFSM_SensorSpec_16_operator/1 -> xxFSM_SensorSpec_18_operator/2
  xxFSM_SensorSpec_17_operator/1 -> xxFSM_SensorSpec_18_operator/1
  xxFSM_SensorSpec_12_operator/1 -> xxFSM_SensorSpec_13_operator/1
  FSM_SensorSpec_MODE/1 -> xxFSM_SensorSpec_10_operator/2
  xxFSM_SensorSpec_9_operator/1 -> xxFSM_SensorSpec_10_operator/1
  xxFSM_SensorSpec_1_operator/1 -> spec203_operator/2
  xxFSM_SensorSpec_6_operator/1 -> spec203_operator/1
  xxFSM_SensorSpec_7_operator/1 -> spec182_operator/2
  xxFSM_SensorSpec_10_operator/1 -> spec182_operator/1
  xxFSM_SensorSpec_11_operator/1 -> spec165_operator/2
  xxFSM_SensorSpec_13_operator/1 -> spec165_operator/1
  xxFSM_SensorSpec_14_operator/1 -> spec151_operator/2
  xxFSM_SensorSpec_19_operator/1 -> spec151_operator/1
  xxFSM_SensorSpec_20_operator/1 -> spec130_operator/2
  xxFSM_SensorSpec_23_operator/1 -> spec130_operator/1
  spec203_operator/1 -> FSM011v2/1(In1)
  spec182_operator/1 -> FSM013/1(In1)
  spec165_operator/1 -> FSM010/1(In1)
  spec151_operator/1 -> FSM012/1(In1)
  spec130_operator/1 -> FSM011v1/1(In1)
  xxFSM_SensorSpec_28_rhs/1 -> xxFSM_SensorSpec_20_operator/2, xxFSM_SensorSpec_1_operator/2, xxFSM_SensorSpec_14_operator/2, xxFSM_SensorSpec_8_operator/2
  FSM_SensorSpec_request/1 -> xxFSM_SensorSpec_9_operator/2, xxFSM_SensorSpec_21_operator/1, xxFSM_SensorSpec_3_operator/1, xxFSM_SensorSpec_16_operator/1
  xxFSM_SensorSpec_26_rhs/1 -> xxFSM_SensorSpec_17_operator/2, xxFSM_SensorSpec_11_operator/2
  FSM_SensorSpec_SENSTATE/1 -> xxFSM_SensorSpec_20_operator/1, xxFSM_SensorSpec_11_operator/1, xxFSM_SensorSpec_7_operator/1, xxFSM_SensorSpec_1_operator/1, xxFSM_SensorSpec_14_operator/1
  FSM_SensorSpec_limits/1 -> xxFSM_SensorSpec_2_operator/1, xxFSM_SensorSpec_15_operator/1, xxFSM_SensorSpec_13_operator/2
  xxFSM_SensorSpec_27_rhs/1 -> xxFSM_SensorSpec_7_operator/2, xxFSM_SensorSpec_22_operator/2, xxFSM_SensorSpec_12_operator/2, xxFSM_SensorSpec_4_operator/2
  FSM_SensorSpec_senstate/1 -> xxFSM_SensorSpec_22_operator/1, xxFSM_SensorSpec_12_operator/1, xxFSM_SensorSpec_4_operator/1, xxFSM_SensorSpec_17_operator/1, xxFSM_SensorSpec_8_operator/1
  FSM011v1/1(guarantee) -> Assertion1/1
  FSM012/1(guarantee) -> Assertion2/1
  FSM010/1(guarantee) -> Assertion3/1
  FSM013/1(guarantee) -> Assertion4/1
  FSM011v2/1(guarantee) -> Assertion5/1

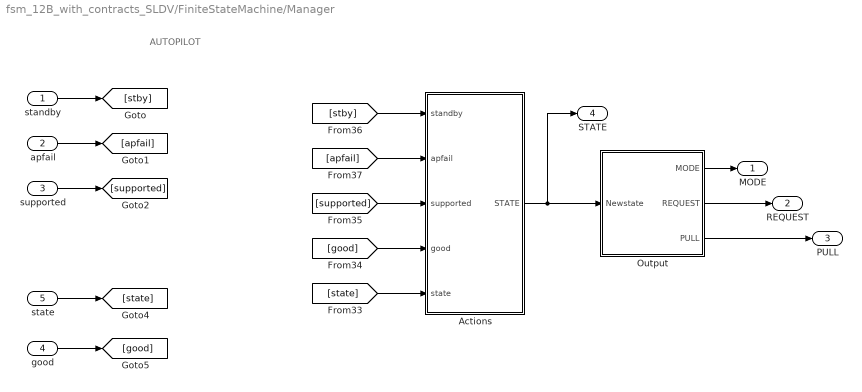
== system fsm_12B_with_contracts_SLDV/FiniteStateMachine/Manager ==
  note: AUTOPILOT
  standby : Inport
  apfail : Inport  Port=2
  supported : Inport  Port=3
  good : Inport  Port=4
  state : Inport  Port=5
  Actions : Subsystem
  Output : Subsystem
  MODE : Outport  VectorParamsAs1DForOutWhenUnconnected=off
  REQUEST : Outport  Port=2  VectorParamsAs1DForOutWhenUnconnected=off
  PULL : Outport  Port=3  VectorParamsAs1DForOutWhenUnconnected=off
  STATE : Outport  Port=4  VectorParamsAs1DForOutWhenUnconnected=off
  wires:
  standby/1 -> [stby]
  supported/1 -> [supported]
  apfail/1 -> [apfail]
  state/1 -> [state]
  good/1 -> [good]
  Actions/1(STATE) -> STATE/1, Output/1(Newstate)
  [apfail] -> Actions/2(apfail)
  [state] -> Actions/5(state)
  [supported] -> Actions/3(supported)
  [good] -> Actions/4(good)
  [stby] -> Actions/1(standby)
  Output/1(MODE) -> MODE/1
  Output/2(REQUEST) -> REQUEST/1
  Output/3(PULL) -> PULL/1

== system fsm_12B_with_contracts_SLDV/FiniteStateMachine/Sen ==
  note: SENSOR
  mode : Inport
  request : Inport  Port=2
  limits : Inport  Port=3
  senstate : Inport  Port=4
  Actions : Subsystem
  Output : Subsystem
  good : Outport  VectorParamsAs1DForOutWhenUnconnected=off
  SENSTATE : Outport  Port=2  VectorParamsAs1DForOutWhenUnconnected=off
  wires:
  request/1 -> [request]
  mode/1 -> [mode]
  limits/1 -> [limits]
  senstate/1 -> [senstate]
  Output/1(Good) -> good/1
  [request] -> Actions/2(request)
  [mode] -> Actions/1(mode)
  Actions/1(SENSTATE) -> Output/1(Newstate), SENSTATE/1
  [senstate] -> Actions/4(senstate)
  [limits] -> Actions/3(limits)

== system fsm_12B_with_contracts_SLDV/fsm_12B_FSMSpec/FSM001v1 ==
  In1 : Inport
  guarantee : Outport  OutDataTypeStr=boolean
  wires:
  In1/1 -> guarantee/1

== system fsm_12B_with_contracts_SLDV/fsm_12B_FSMSpec/FSM001v2 ==
  In1 : Inport
  guarantee : Outport  OutDataTypeStr=boolean
  wires:
  In1/1 -> guarantee/1

== system fsm_12B_with_contracts_SLDV/fsm_12B_FSMSpec/FSM001v3 ==
  In1 : Inport
  guarantee : Outport  OutDataTypeStr=boolean
  wires:
  In1/1 -> guarantee/1

== system fsm_12B_with_contracts_SLDV/fsm_12B_FSMSpec/HT_call ==
  HT_L : Inport
  HT_R : Inport  Port=2
  HT_X : Inport  Port=3  OutDataTypeStr=boolean
  OT_call : Subsystem
  Y_operator : Logic  Operator=NOT  AllPortsSameDT=off  OutDataTypeStr=boolean
  xxHT_1_operator : Logic  Operator=NOT  AllPortsSameDT=off  OutDataTypeStr=boolean
  HT_Y : Outport
  wires:
  Y_operator/1 -> HT_Y/1
  HT_X/1 -> xxHT_1_operator/1
  OT_call/1(OT_Y) -> Y_operator/1
  xxHT_1_operator/1 -> OT_call/3(OT_X)
  HT_R/1 -> OT_call/2(OT_R)
  HT_L/1 -> OT_call/1(OT_L)

== system fsm_12B_with_contracts_SLDV/fsm_12B_FSMSpec/HT_call1 ==
  HT_L : Inport
  HT_R : Inport  Port=2
  HT_X : Inport  Port=3  OutDataTypeStr=boolean
  OT_call : Subsystem
  Y_operator : Logic  Operator=NOT  AllPortsSameDT=off  OutDataTypeStr=boolean
  xxHT_1_operator : Logic  Operator=NOT  AllPortsSameDT=off  OutDataTypeStr=boolean
  HT_Y : Outport
  wires:
  Y_operator/1 -> HT_Y/1
  HT_X/1 -> xxHT_1_operator/1
  OT_call/1(OT_Y) -> Y_operator/1
  xxHT_1_operator/1 -> OT_call/3(OT_X)
  HT_R/1 -> OT_call/2(OT_R)
  HT_L/1 -> OT_call/1(OT_L)

== system fsm_12B_with_contracts_SLDV/FiniteStateMachine/FiniteStateMachine_FSM_AutopilotSpec1/FSM002 ==
  In1 : Inport
  guarantee : Outport  OutDataTypeStr=boolean
  wires:
  In1/1 -> guarantee/1

== system fsm_12B_with_contracts_SLDV/FiniteStateMachine/FiniteStateMachine_FSM_AutopilotSpec1/FSM003 ==
  In1 : Inport
  guarantee : Outport  OutDataTypeStr=boolean
  wires:
  In1/1 -> guarantee/1

== system fsm_12B_with_contracts_SLDV/FiniteStateMachine/FiniteStateMachine_FSM_AutopilotSpec1/FSM003v2 ==
  In1 : Inport
  guarantee : Outport  OutDataTypeStr=boolean
  wires:
  In1/1 -> guarantee/1

== system fsm_12B_with_contracts_SLDV/FiniteStateMachine/FiniteStateMachine_FSM_AutopilotSpec1/FSM004 ==
  In1 : Inport
  guarantee : Outport  OutDataTypeStr=boolean
  wires:
  In1/1 -> guarantee/1

== system fsm_12B_with_contracts_SLDV/FiniteStateMachine/FiniteStateMachine_FSM_AutopilotSpec1/FSM004v2 ==
  In1 : Inport
  guarantee : Outport  OutDataTypeStr=boolean
  wires:
  In1/1 -> guarantee/1

== system fsm_12B_with_contracts_SLDV/FiniteStateMachine/FiniteStateMachine_FSM_AutopilotSpec1/FSM005 ==
  In1 : Inport
  guarantee : Outport  OutDataTypeStr=boolean
  wires:
  In1/1 -> guarantee/1

== system fsm_12B_with_contracts_SLDV/FiniteStateMachine/FiniteStateMachine_FSM_AutopilotSpec1/FSM006 ==
  In1 : Inport
  guarantee : Outport  OutDataTypeStr=boolean
  wires:
  In1/1 -> guarantee/1

== system fsm_12B_with_contracts_SLDV/FiniteStateMachine/FiniteStateMachine_FSM_AutopilotSpec1/FSM007 ==
  In1 : Inport
  guarantee : Outport  OutDataTypeStr=boolean
  wires:
  In1/1 -> guarantee/1

== system fsm_12B_with_contracts_SLDV/FiniteStateMachine/FiniteStateMachine_FSM_AutopilotSpec1/FSM007v2 ==
  In1 : Inport
  guarantee : Outport  OutDataTypeStr=boolean
  wires:
  In1/1 -> guarantee/1

== system fsm_12B_with_contracts_SLDV/FiniteStateMachine/FiniteStateMachine_FSM_AutopilotSpec1/FSM008v1 ==
  In1 : Inport
  guarantee : Outport  OutDataTypeStr=boolean
  wires:
  In1/1 -> guarantee/1

== system fsm_12B_with_contracts_SLDV/FiniteStateMachine/FiniteStateMachine_FSM_AutopilotSpec1/FSM008v2 ==
  In1 : Inport
  guarantee : Outport  OutDataTypeStr=boolean
  wires:
  In1/1 -> guarantee/1

== system fsm_12B_with_contracts_SLDV/FiniteStateMachine/FiniteStateMachine_FSM_AutopilotSpec1/FSM009 ==
  In1 : Inport
  guarantee : Outport  OutDataTypeStr=boolean
  wires:
  In1/1 -> guarantee/1

== system fsm_12B_with_contracts_SLDV/FiniteStateMachine/FiniteStateMachine_FSM_SensorSpec/FSM010 ==
  In1 : Inport
  guarantee : Outport  OutDataTypeStr=boolean
  wires:
  In1/1 -> guarantee/1

== system fsm_12B_with_contracts_SLDV/FiniteStateMachine/FiniteStateMachine_FSM_SensorSpec/FSM011v1 ==
  In1 : Inport
  guarantee : Outport  OutDataTypeStr=boolean
  wires:
  In1/1 -> guarantee/1

== system fsm_12B_with_contracts_SLDV/FiniteStateMachine/FiniteStateMachine_FSM_SensorSpec/FSM011v2 ==
  In1 : Inport
  guarantee : Outport  OutDataTypeStr=boolean
  wires:
  In1/1 -> guarantee/1

== system fsm_12B_with_contracts_SLDV/FiniteStateMachine/FiniteStateMachine_FSM_SensorSpec/FSM012 ==
  In1 : Inport
  guarantee : Outport  OutDataTypeStr=boolean
  wires:
  In1/1 -> guarantee/1

== system fsm_12B_with_contracts_SLDV/FiniteStateMachine/FiniteStateMachine_FSM_SensorSpec/FSM013 ==
  In1 : Inport
  guarantee : Outport  OutDataTypeStr=boolean
  wires:
  In1/1 -> guarantee/1

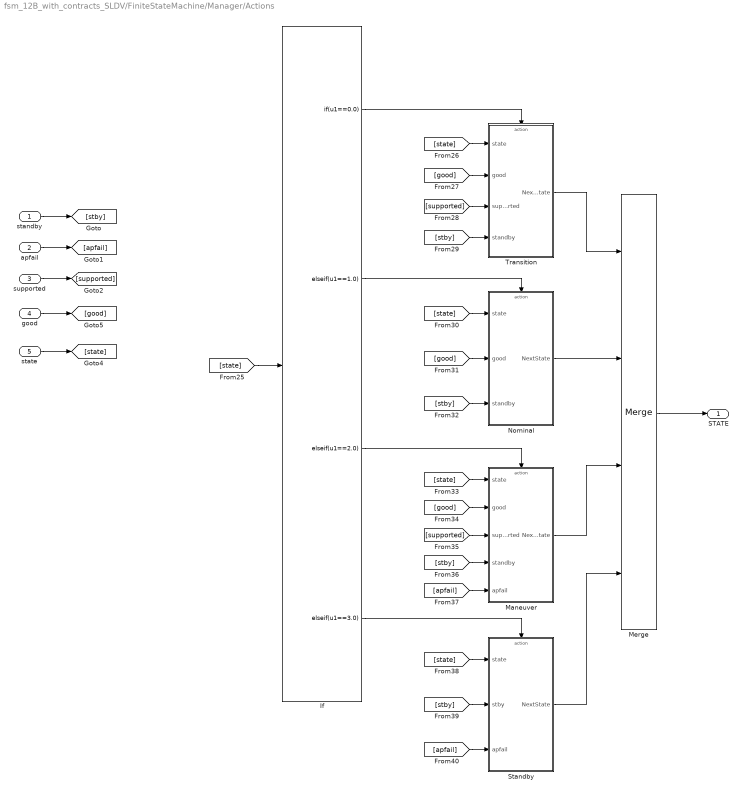
== system fsm_12B_with_contracts_SLDV/FiniteStateMachine/Manager/Actions ==
  standby : Inport
  apfail : Inport  Port=2
  supported : Inport  Port=3
  good : Inport  Port=4
  state : Inport  Port=5
  If : If  IfExpression=u1==0.0  ElseIfExpressions=u1==1.0, u1==2.0, u1==3.0  ShowElse=off
  Maneuver : Subsystem
  Merge : Merge  Inputs=4
  Nominal : Subsystem
  Standby : Subsystem
  Transition : Subsystem
  STATE : Outport  VectorParamsAs1DForOutWhenUnconnected=off
  wires:
  [state] -> If/1
  [state] -> Transition/1(state)
  [apfail] -> Standby/3(apfail)
  [stby] -> Standby/2(stby)
  Standby/1(NextState) -> Merge/4
  [state] -> Standby/1(state)
  Maneuver/1(NextState) -> Merge/3
  Merge/1 -> STATE/1
  Transition/1(NextState) -> Merge/1
  Nominal/1(NextState) -> Merge/2
  If/2 -> Nominal/Action
  [state] -> Nominal/1(state)
  If/3 -> Maneuver/Action
  If/4 -> Standby/Action
  [apfail] -> Maneuver/5(apfail)
  [good] -> Nominal/2(good)
  [stby] -> Nominal/3(standby)
  If/1 -> Transition/Action
  [supported] -> Transition/3(supported)
  [good] -> Transition/2(good)
  [stby] -> Transition/4(standby)
  [state] -> Maneuver/1(state)
  [supported] -> Maneuver/3(supported)
  [good] -> Maneuver/2(good)
  [stby] -> Maneuver/4(standby)
  standby/1 -> [stby]
  supported/1 -> [supported]
  apfail/1 -> [apfail]
  state/1 -> [state]
  good/1 -> [good]

== system fsm_12B_with_contracts_SLDV/FiniteStateMachine/Manager/Output ==
  Newstate : Inport
  Demux : Demux  Outputs=3
  If : If  IfExpression=u1==0.0  ElseIfExpressions=u1==1.0, u1==2.0, u1==3.0  ShowElse=off
  Maneuver : Subsystem
  Merge : Merge  Inputs=4
  Nominal : Subsystem
  Standby : Subsystem
  Transition : Subsystem
  MODE : Outport  VectorParamsAs1DForOutWhenUnconnected=off
  REQUEST : Outport  Port=2  VectorParamsAs1DForOutWhenUnconnected=off
  PULL : Outport  Port=3  VectorParamsAs1DForOutWhenUnconnected=off
  wires:
  Demux/2 -> REQUEST/1  "REQUEST"
  Demux/1 -> MODE/1  "MODE"
  Demux/3 -> PULL/1  "PULL"
  Merge/1 -> Demux/1
  Nominal/1(Output) -> Merge/2
  Maneuver/1(Output) -> Merge/3
  If/2 -> Nominal/Action
  Transition/1(Output) -> Merge/1
  If/3 -> Maneuver/Action
  Standby/1(Output) -> Merge/4
  If/1 -> Transition/Action
  Newstate/1 -> If/1
  If/4 -> Standby/Action

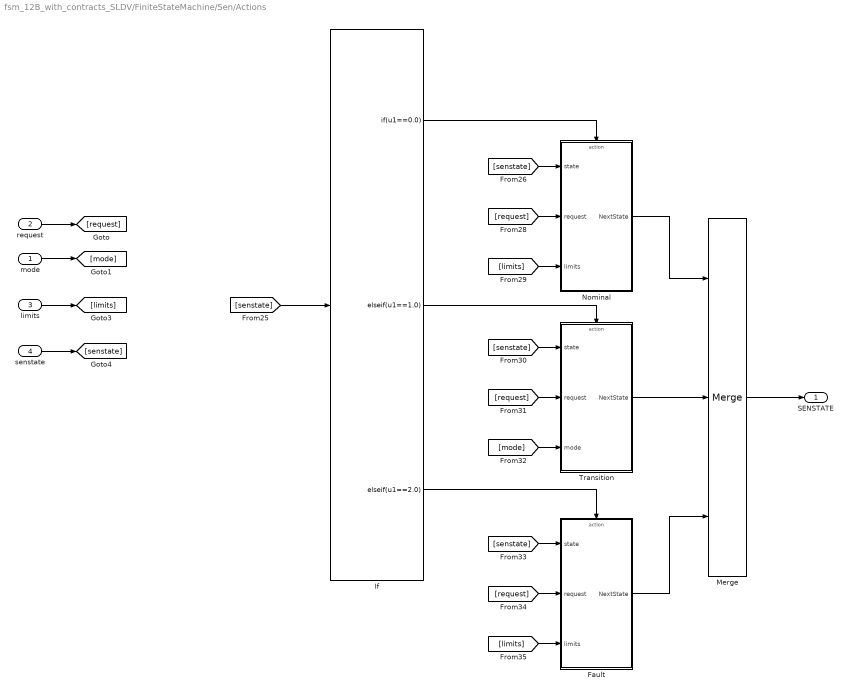
== system fsm_12B_with_contracts_SLDV/FiniteStateMachine/Sen/Actions ==
  mode : Inport
  request : Inport  Port=2
  limits : Inport  Port=3
  senstate : Inport  Port=4
  Fault : Subsystem
  If : If  IfExpression=u1==0.0  ElseIfExpressions=u1==1.0, u1==2.0  ShowElse=off
  Merge : Merge  Inputs=3
  Nominal : Subsystem
  Transition : Subsystem
  SENSTATE : Outport  VectorParamsAs1DForOutWhenUnconnected=off
  wires:
  [senstate] -> If/1
  [senstate] -> Nominal/1(state)
  Fault/1(NextState) -> Merge/3
  Merge/1 -> SENSTATE/1
  Nominal/1(NextState) -> Merge/1
  Transition/1(NextState) -> Merge/2
  If/2 -> Transition/Action
  [senstate] -> Transition/1(state)
  If/3 -> Fault/Action
  [request] -> Transition/2(request)
  [mode] -> Transition/3(mode)
  If/1 -> Nominal/Action
  [request] -> Nominal/2(request)
  [limits] -> Nominal/3(limits)
  [senstate] -> Fault/1(state)
  [limits] -> Fault/3(limits)
  [request] -> Fault/2(request)
  request/1 -> [request]
  mode/1 -> [mode]
  limits/1 -> [limits]
  senstate/1 -> [senstate]

== system fsm_12B_with_contracts_SLDV/FiniteStateMachine/Sen/Output ==
  Newstate : Inport
  Constant12 : Constant  OutDataTypeStr=boolean
  Constant6 : Constant  Value=2
  Constant9 : Constant  Value=0  OutDataTypeStr=boolean
  Relational Operator5 : RelationalOperator  Operator===  OutDataTypeStr=boolean  RndMeth=Nearest
  Switch2 : Switch  Criteria=u2 ~= 0
  Good : Outport  VectorParamsAs1DForOutWhenUnconnected=off
  wires:
  Constant6/1 -> Relational Operator5/2
  Relational Operator5/1 -> Switch2/2
  Constant9/1 -> Switch2/1
  Constant12/1 -> Switch2/3
  Switch2/1 -> Good/1
  Newstate/1 -> Relational Operator5/1

== system fsm_12B_with_contracts_SLDV/fsm_12B_FSMSpec/HT_call/OT_call ==
  OT_L : Inport
  OT_R : Inport  Port=2
  OT_X : Inport  Port=3  OutDataTypeStr=boolean
  OTlore_call : Subsystem
  delay_call : Subsystem
  xxOT_1_operator : Sum  Inputs=+-  OutDataTypeStr=int32
  OT_Y : Outport
  wires:
  OTlore_call/1(OTlore_Y) -> OT_Y/1
  OT_L/1 -> xxOT_1_operator/1
  OT_X/1 -> delay_call/1(delay_X)
  delay_call/1(delay_Y) -> OTlore_call/2(OTlore_X)
  xxOT_1_operator/1 -> OTlore_call/1(OTlore_N)
  OT_R/1 -> xxOT_1_operator/2, delay_call/2(delay_R)

== system fsm_12B_with_contracts_SLDV/fsm_12B_FSMSpec/HT_call1/OT_call ==
  OT_L : Inport
  OT_R : Inport  Port=2
  OT_X : Inport  Port=3  OutDataTypeStr=boolean
  OTlore_call : Subsystem
  delay_call : Subsystem
  xxOT_1_operator : Sum  Inputs=+-  OutDataTypeStr=int32
  OT_Y : Outport
  wires:
  OTlore_call/1(OTlore_Y) -> OT_Y/1
  OT_L/1 -> xxOT_1_operator/1
  OT_X/1 -> delay_call/1(delay_X)
  delay_call/1(delay_Y) -> OTlore_call/2(OTlore_X)
  xxOT_1_operator/1 -> OTlore_call/1(OTlore_N)
  OT_R/1 -> xxOT_1_operator/2, delay_call/2(delay_R)

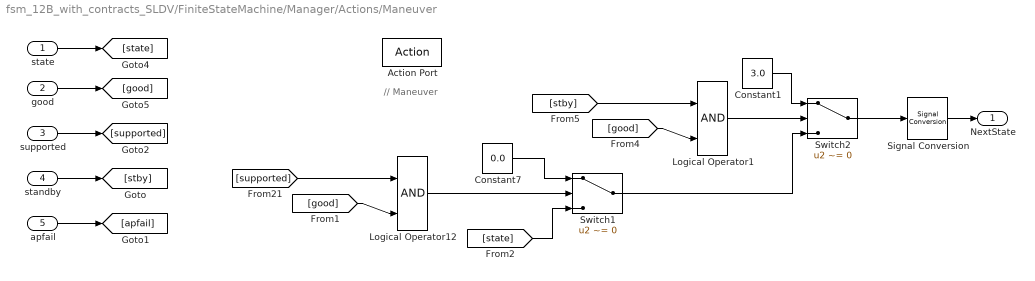
== system fsm_12B_with_contracts_SLDV/FiniteStateMachine/Manager/Actions/Maneuver ==
  note: // Maneuver
  state : Inport
  good : Inport  Port=2
  supported : Inport  Port=3
  standby : Inport  Port=4
  apfail : Inport  Port=5
  Action Port : ActionPort  ActionPortLabel=elseif( u1==2.0)
  Constant1 : Constant  Value=3.0
  Constant7 : Constant  Value=0.0
  Logical Operator1 : Logic  IconShape=distinctive  AllPortsSameDT=off  OutDataTypeStr=boolean
  Logical Operator12 : Logic  IconShape=distinctive  AllPortsSameDT=off  OutDataTypeStr=boolean
  Signal Conversion : SignalConversion  OverrideOpt=off
  Switch1 : Switch  Criteria=u2 ~= 0
  Switch2 : Switch  Criteria=u2 ~= 0
  NextState : Outport  VectorParamsAs1DForOutWhenUnconnected=off
  wires:
  [supported] -> Logical Operator12/1
  Logical Operator12/1 -> Switch1/2
  [state] -> Switch1/3
  Constant7/1 -> Switch1/1
  Logical Operator1/1 -> Switch2/2
  Constant1/1 -> Switch2/1
  Switch2/1 -> Signal Conversion/1
  Signal Conversion/1 -> NextState/1
  standby/1 -> [stby]
  supported/1 -> [supported]
  apfail/1 -> [apfail]
  state/1 -> [state]
  good/1 -> [good]
  [good] -> Logical Operator12/2
  [stby] -> Logical Operator1/1
  [good] -> Logical Operator1/2
  Switch1/1 -> Switch2/3

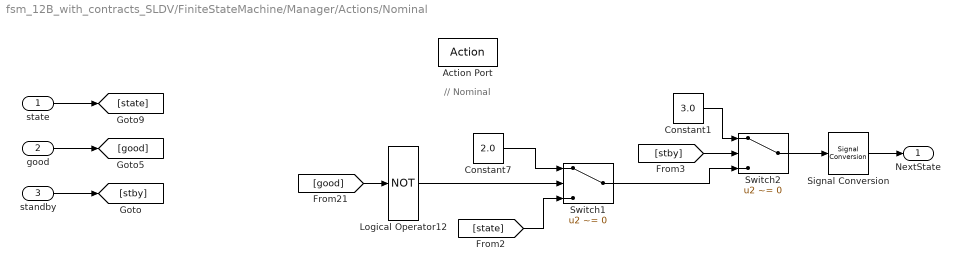
== system fsm_12B_with_contracts_SLDV/FiniteStateMachine/Manager/Actions/Nominal ==
  note: // Nominal
  state : Inport
  good : Inport  Port=2
  standby : Inport  Port=3
  Action Port : ActionPort  ActionPortLabel=elseif(u1==1.0)
  Constant1 : Constant  Value=3.0
  Constant7 : Constant  Value=2.0
  Logical Operator12 : Logic  Operator=NOT  IconShape=distinctive  AllPortsSameDT=off  OutDataTypeStr=boolean
  Signal Conversion : SignalConversion  OverrideOpt=off
  Switch1 : Switch  Criteria=u2 ~= 0
  Switch2 : Switch  Criteria=u2 ~= 0
  NextState : Outport  VectorParamsAs1DForOutWhenUnconnected=off
  wires:
  Signal Conversion/1 -> NextState/1
  Switch2/1 -> Signal Conversion/1
  Switch1/1 -> Switch2/3
  Constant1/1 -> Switch2/1
  [stby] -> Switch2/2
  standby/1 -> [stby]
  Constant7/1 -> Switch1/1
  [state] -> Switch1/3
  Logical Operator12/1 -> Switch1/2
  [good] -> Logical Operator12/1
  good/1 -> [good]
  state/1 -> [state]
